simulink model "CH13_2E"  (Simulink 10.0)
settings: Solver=ode45  StartTime=0.0  StopTime=1e-4  RelTol=1e-3
libraries: commsynccomp2 x2, dsparch4 x1
settings Model: Creator=my2  LastModifiedBy=IT
settings DataIOCC: LimitDataPoints=on  SignalLoggingSaveFormat=ModelDataLogs
settings OptimizationCC: BlockReduction=off  BooleanDataType=off
settings DebuggingCC: SaveWithParameterizedLinksMsg=none  SignalResolutionControl=TryResolveAllWithWarning  FcnCallInpInsideContextMsg=warning
settings HardwareCC: TargetUnknown=on
settings GRTTargetCC: GeneratePreprocessorConditionals=Disable all
settings ConfigComp: CovExternalEMLEnable=off

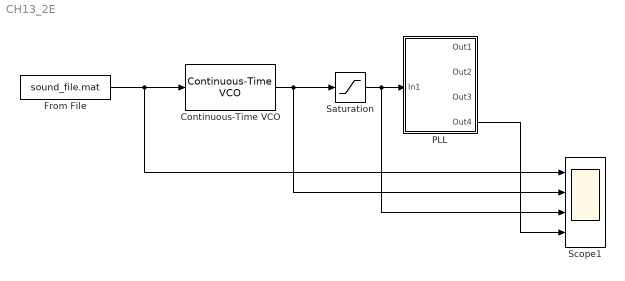
== system CH13_2E ==
  Continuous-Time VCO : commsynccomp2/Continuous-Time VCO  Ac=1  Fc=10  Kc=1  Ph=0
      settings: SourceProductName=Communications Toolbox  SourceProductBaseCode=CM
  From File : FromFile  FileName=sound_file.mat  SampleTime=0
  PLL : Subsystem
  Saturation : Saturate
  Scope1 : Scope  NumInputPorts=4
  wires:
  From File/1 -> Continuous-Time VCO/1, Scope1/1
  Continuous-Time VCO/1 -> Saturation/1, Scope1/2
  Saturation/1 -> Scope1/3, PLL/1(In1)
  PLL/4(Out4) -> Scope1/4

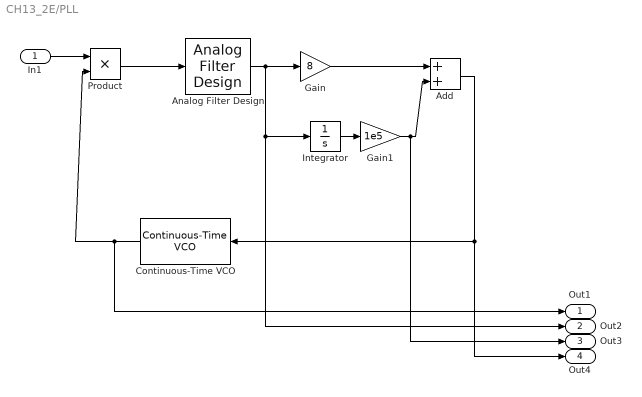
== system CH13_2E/PLL ==
  In1 : Inport
  Add : Sum
  Analog Filter Design : dsparch4/Analog Filter Design  method=Chebyshev II  filttype=Lowpass  N=32  Wlo=2*pi*50e3  Whi=80  Rp=2  Rs=40
  Continuous-Time VCO : commsynccomp2/Continuous-Time VCO  Ac=1  Fc=93e3  Kc=1000  Ph=0
      settings: SourceProductName=Communications Toolbox  SourceProductBaseCode=CM
  Gain : Gain  Gain=8
  Gain1 : Gain  Gain=1e5
  Integrator : Integrator
  Product : Product
  Out1 : Outport
  Out2 : Outport  Port=2
  Out3 : Outport  Port=3
  Out4 : Outport  Port=4
  wires:
  In1/1 -> Product/1
  Add/1 -> Out4/1, Continuous-Time VCO/1
  Product/1 -> Analog Filter Design/1
  Analog Filter Design/1 -> Out2/1, Integrator/1, Gain/1
  Integrator/1 -> Gain1/1
  Gain/1 -> Add/1
  Gain1/1 -> Out3/1, Add/2
  Continuous-Time VCO/1 -> Out1/1, Product/2
